simulink subsystem "Recevoir_les_pieces"  (R2020a)
settings: Solver=VariableStepAuto  StartTime=0.0  StopTime=10.0  RelTol=1e-3
settings Model: Creator=frfoc1  LastModifiedBy=frfoc1

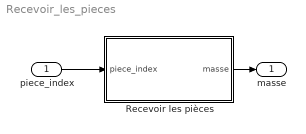
== system Recevoir_les_pieces ==
  piece_index : Inport
  Recevoir les pièces : MATLAB Function  TreatAsAtomicUnit=on
  masse : Outport
  wires:
  piece_index/1 -> Recevoir les pièces/1(piece_index)
  Recevoir les pièces/1(masse) -> masse/1

== matlab function Recevoir_les_pieces/Recevoir les pièces ==
  data: piece_index input; masse output
function masse = get_masse_piece(piece_index)
    if piece_index == 0
        masse = 3.950; % 5 cents
    elseif piece_index == 1
        masse = 1.750; % 10 cents
    elseif piece_index == 2
        masse = 4.400; % 25 cents
    elseif piece_index == 3
        masse = 6.270; % 1 dollar
    elseif piece_index == 4
        masse = 6.920; % 2 dollar
    else
        disp("Pièce invalide");
        masse = 0;
    end
